simulink model "FT_CAN_Test"  (R2021b)
settings: Solver=FixedStepDiscrete  StartTime=0.0  StopTime=Inf  RelTol=1e-3
undefined symbols (not defined in the file): canChannel
libraries: canmsglib x10, canlib x4
settings Model: Creator=mfussi  LastModifiedBy=mfussi

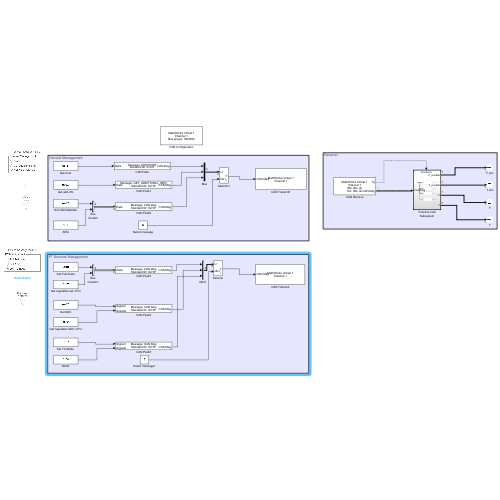
[thumbnail: Simulink's stored preview of the top-level diagram]
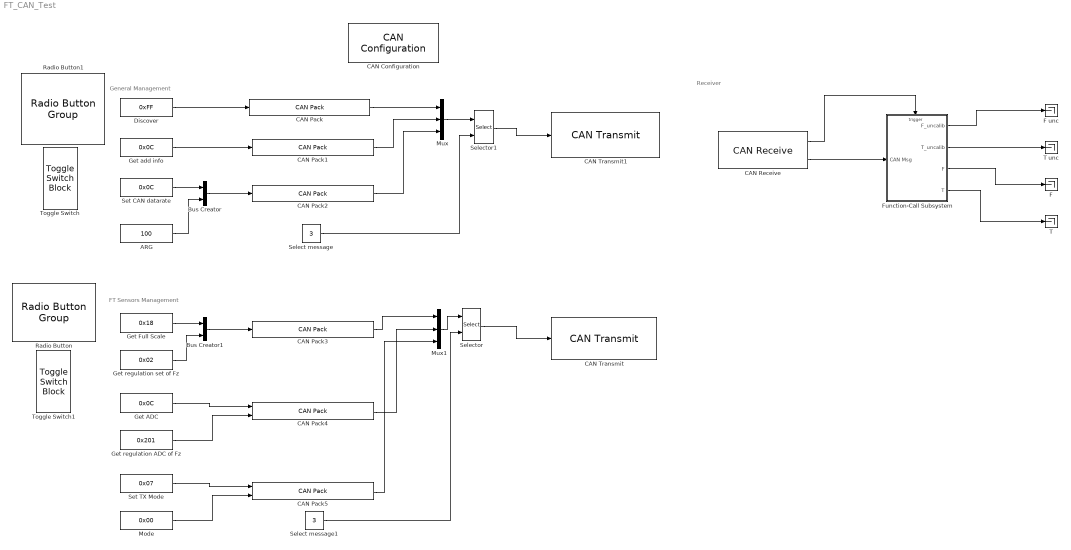
== system FT_CAN_Test ==
  note: Receiver
  note: FT Sensors Management
  note: General Management
  ARG : Constant  Value=100  OutDataTypeStr=uint8
  Bus Creator : BusCreator  Inputs=2
  Bus Creator1 : BusCreator  Inputs=2
  CAN Configuration : canlib/CAN Configuration  BlockHandle=6.0001  Device=MathWorks Virtual 1 (Channel 1)  DeviceMenu=MathWorks Virtual 1 (Channel 1)  ObjConstructor=canChannel('MathWorks', 'Virtual 1', 1)  BusSpeed=1000000  EnableBitParameters=off  AckMode=Normal
      settings: SourceProductBaseCode=VN
  CAN Pack : canmsglib/CAN Pack  MsgList=(none)  MsgName=DISCOVER  MsgIDType=Standard (11-bit identifier)  MsgIdentifier=0x70F  MsgLength=1  Remote=off  ApplyMinMax=off  BusOutput=off  SignalInfo={}
      settings: SourceProductBaseCode=ME,XP,VN  DataFormat=raw data
  CAN Pack1 : canmsglib/CAN Pack  MsgList=(none)  MsgName=GET_ADDITIONAL_INFO  MsgIDType=Standard (11-bit identifier)  MsgIdentifier=0x70F  MsgLength=1  Remote=off  ApplyMinMax=off  BusOutput=off  SignalInfo={}
      settings: SourceProductBaseCode=ME,XP,VN  DataFormat=raw data
  CAN Pack2 : canmsglib/CAN Pack  MsgList=(none)  MsgName=CAN Msg  MsgIDType=Standard (11-bit identifier)  MsgIdentifier=0x70F  MsgLength=1  Remote=off  ApplyMinMax=off  BusOutput=off  SignalInfo={}
      settings: SourceProductBaseCode=ME,XP,VN  DataFormat=raw data
  CAN Pack3 : canmsglib/CAN Pack  MsgList=(none)  MsgName=CAN Msg  MsgIDType=Standard (11-bit identifier)  MsgIdentifier=0x70F  MsgLength=2  Remote=off  ApplyMinMax=off  BusOutput=off  SignalInfo={}
      settings: SourceProductBaseCode=ME,XP,VN  DataFormat=raw data
  CAN Pack4 : canmsglib/CAN Pack  MsgList=(none)  MsgName=CAN Msg  MsgIDType=Standard (11-bit identifier)  MsgIdentifier=0x70F  MsgLength=3  Remote=off  ApplyMinMax=off  BusOutput=off  SignalInfo={ 'Signal1', '0', '8', 'LE', 'unsigned', 'Standard', '0', '1', '0', '-Inf', 'Inf'; 'Signal2', '8', '16', 'LE', 'unsigned', 'Standard', '0', '1', '0', '-Inf', 'Inf' }
      settings: SourceProductBaseCode=ME,XP,VN  DataFormat=manually specified signals
  CAN Pack5 : canmsglib/CAN Pack  MsgList=(none)  MsgName=CAN Msg  MsgIDType=Standard (11-bit identifier)  MsgIdentifier=0x70F  MsgLength=2  Remote=off  ApplyMinMax=off  BusOutput=off  SignalInfo={ 'Signal1', '0', '8', 'LE', 'unsigned', 'Standard', '0', '1', '0', '-Inf', 'Inf'; 'Signal2', '8', '8', 'LE', 'unsigned', 'Standard', '0', '1', '0', '-Inf', 'Inf' }
      settings: SourceProductBaseCode=ME,XP,VN  DataFormat=manually specified signals
  CAN Receive : canlib/CAN Receive  BlockHandle=12.0001  Device=MathWorks Virtual 1 (Channel 1)  DeviceMenu=MathWorks Virtual 1 (Channel 1)  ObjConstructor=canChannel('MathWorks', 'Virtual 1', 1)  EnableStandardIDsFilter=off  StdIDsCombo=Allow all  StandardIDs=0  EnableExtendedIDsFilter=off  ExtIDsCombo=Allow all  ExtendedIDs=0  SampleTime=0.01  MsgsPerTimestep=all  InternalFilterUpdateStatus=on  BusOutput=on
      settings: SourceProductBaseCode=VN
  CAN Transmit : canlib/CAN Transmit  BlockHandle=13.0001  Device=MathWorks Virtual 1 (Channel 1)  DeviceMenu=MathWorks Virtual 1 (Channel 1)  ObjConstructor=canChannel('MathWorks', 'Virtual 1', 1)  EnableEventTransmit=off  EnablePeriodicTransmit=off  MessagePeriod=1.000
      settings: SourceProductBaseCode=VN
  CAN Transmit1 : canlib/CAN Transmit  BlockHandle=13.0001  Device=MathWorks Virtual 1 (Channel 1)  DeviceMenu=MathWorks Virtual 1 (Channel 1)  ObjConstructor=canChannel('MathWorks', 'Virtual 1', 1)  EnableEventTransmit=off  EnablePeriodicTransmit=off  MessagePeriod=1.000
      settings: SourceProductBaseCode=VN
  Discover : Constant  Value=0xFF
  F : Terminator
  F unc : Terminator
  Function-Call Subsystem : Subsystem  TreatAsAtomicUnit=on
  Get ADC : Constant  Value=0x0C  OutDataTypeStr=uint8
  Get Full Scale : Constant  Value=0x18  OutDataTypeStr=uint8
  Get add info : Constant  Value=0x0C
  Get regulation ADC of Fz : Constant  Value=0x201  OutDataTypeStr=uint16
  Get regulation set of Fz : Constant  Value=0x02  OutDataTypeStr=uint8
  Mode : Constant  Value=0x00  OutDataTypeStr=uint8
  Mux : Mux  Inputs=3
  Mux1 : Mux  Inputs=3
  Radio Button : RadioButtonGroup  SelectedLabel=Set TX mode  ButtonGroupName=FT Management
      settings: Values={{'Get Full scale', 'Get ADC', 'Set TX mode'}, [1 2 3]}
  Radio Button1 : RadioButtonGroup  SelectedLabel=Set CAN datarate  ButtonGroupName=General Management
      settings: Values={{'Discover', 'Get additional info', 'Set CAN datarate'}, [1 2 3]}
  Select message : Constant  Value=3
  Select message1 : Constant  Value=3
  Selector : Selector  InputPortWidth=3  IndexOptions=Index vector (port)  Indices=[1 3]  OutputSizes=1
  Selector1 : Selector  InputPortWidth=3  IndexOptions=Index vector (port)  Indices=[1 3]  OutputSizes=1
  Set CAN datarate : Constant  Value=0x0C
  "Set TX Mode " : Constant  Value=0x07
  T : Terminator
  T unc : Terminator
  Toggle Switch : ToggleSwitchBlock
      settings: Values={{'Off', 'On'}, [0 1]}
  Toggle Switch1 : ToggleSwitchBlock
      settings: Values={{'Off', 'On'}, [0 1]}
  wires:
  Discover/1 -> CAN Pack/1
  CAN Receive/1 -> Function-Call Subsystem/Trigger
  CAN Receive/2 -> Function-Call Subsystem/1(CAN Msg)
  Set CAN datarate/1 -> Bus Creator/1
  ARG/1 -> Bus Creator/2
  Get Full Scale/1 -> Bus Creator1/1
  Get regulation set of Fz/1 -> Bus Creator1/2
  Get add info/1 -> CAN Pack1/1
  CAN Pack1/1 -> Mux/2
  Bus Creator1/1 -> CAN Pack3/1
  CAN Pack2/1 -> Mux/3
  Bus Creator/1 -> CAN Pack2/1
  CAN Pack/1 -> Mux/1
  Get ADC/1 -> CAN Pack4/1
  Get regulation ADC of Fz/1 -> CAN Pack4/2
  "Set TX Mode "/1 -> CAN Pack5/1
  Mode/1 -> CAN Pack5/2
  CAN Pack3/1 -> Mux1/1
  CAN Pack4/1 -> Mux1/2
  CAN Pack5/1 -> Mux1/3
  Mux1/1 -> Selector/1
  Select message1/1 -> Selector/2
  Function-Call Subsystem/1(F_uncalib) -> F unc/1
  Function-Call Subsystem/2(T_uncalib) -> T unc/1
  Function-Call Subsystem/3(F) -> F/1
  Function-Call Subsystem/4(T) -> T/1
  Selector1/1 -> CAN Transmit1/1
  Selector/1 -> CAN Transmit/1
  Select message/1 -> Selector1/2
  Mux/1 -> Selector1/1

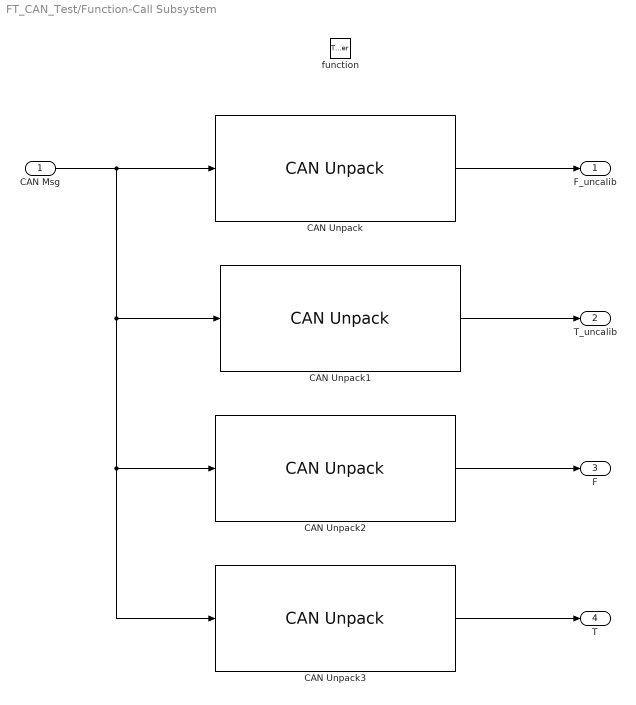
== system FT_CAN_Test/Function-Call Subsystem ==
  CAN Msg : Inport
  function : TriggerPort  TriggerType=function-call  VariantControl=(inherit)
  CAN Unpack : canmsglib/CAN Unpack  MsgList=(none)  MsgName=UNCALIB_F_VECT_DBM  MsgIDType=Standard (11-bit identifier)  MsgIdentifier=1824  MsgLength=7  SignalInfo={}  IDPort=off  TimestampPort=off  ErrorPort=off  RemotePort=off  LengthPort=off  StatusPort=off  ApplyMinMax=off
      settings: SourceProductBaseCode=ME,XP,VN  DataFormat=raw data
  CAN Unpack1 : canmsglib/CAN Unpack  MsgList=(none)  MsgName=UNCALIB_T_VECT_DBM  MsgIDType=Standard (11-bit identifier)  MsgIdentifier=1824  MsgLength=7  SignalInfo={}  IDPort=off  TimestampPort=off  ErrorPort=off  RemotePort=off  LengthPort=off  StatusPort=off  ApplyMinMax=off
      settings: SourceProductBaseCode=ME,XP,VN  DataFormat=raw data
  CAN Unpack2 : canmsglib/CAN Unpack  MsgList=(none)  MsgName=FORCE_VECT  MsgIDType=Standard (11-bit identifier)  MsgIdentifier=1824  MsgLength=7  SignalInfo={}  IDPort=off  TimestampPort=off  ErrorPort=off  RemotePort=off  LengthPort=off  StatusPort=off  ApplyMinMax=off
      settings: SourceProductBaseCode=ME,XP,VN  DataFormat=raw data
  CAN Unpack3 : canmsglib/CAN Unpack  MsgList=(none)  MsgName=FORCE_VECT  MsgIDType=Standard (11-bit identifier)  MsgIdentifier=1824  MsgLength=7  SignalInfo={}  IDPort=off  TimestampPort=off  ErrorPort=off  RemotePort=off  LengthPort=off  StatusPort=off  ApplyMinMax=off
      settings: SourceProductBaseCode=ME,XP,VN  DataFormat=raw data
  F_uncalib : Outport
  T_uncalib : Outport  Port=2
  F : Outport  Port=3
  T : Outport  Port=4
  wires:
  CAN Msg/1 -> CAN Unpack3/1, CAN Unpack2/1, CAN Unpack1/1, CAN Unpack/1
  CAN Unpack/1 -> F_uncalib/1
  CAN Unpack1/1 -> T_uncalib/1
  CAN Unpack2/1 -> F/1
  CAN Unpack3/1 -> T/1
